simulink model "WorkerProductivity"  (R2024b)
settings: Solver=FixedStepAuto  StartTime=0.0  StopTime=100.0  FixedStep=0.01  RelTol=1e-3
settings Model: Creator=max  LastModifiedBy=max

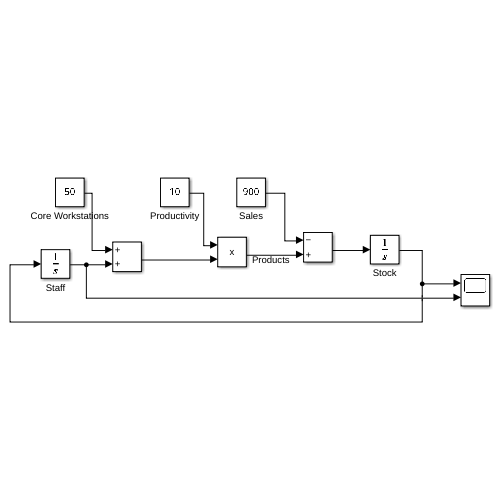
[thumbnail: Simulink's stored preview of the top-level diagram]
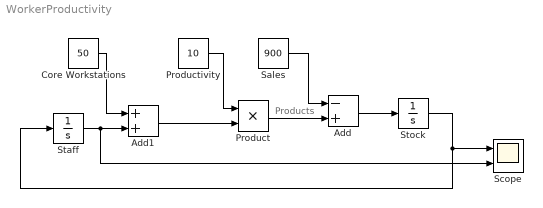
== system WorkerProductivity ==
  note: Products
  Add : Sum  Inputs=-+
  Add1 : Sum
  Core Workstations : Constant  Value=50
  Product : Product
  Productivity : Constant  Value=10
  Sales : Constant  Value=900
  Scope : Scope  NumInputPorts=2
  Staff : Integrator
  Stock : Integrator  InitialCondition=100
  wires:
  Add/1 -> Stock/1
  Sales/1 -> Add/1
  Product/1 -> Add/2
  Productivity/1 -> Product/1
  Stock/1 -> Staff/1, Scope/1
  Staff/1 -> Scope/2, Add1/2
  Add1/1 -> Product/2
  Core Workstations/1 -> Add1/1
